simulink model "InnerTransitiontoJunction"  (R2020b)
settings: Solver=VariableStepAuto  StartTime=0.0  StopTime=10.0  RelTol=1e-3
settings Model: Creator=apple  LastModifiedBy=apple

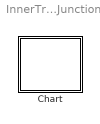
== system InnerTransitiontoJunction ==
  Chart : Stateflow chart  TreatAsAtomicUnit=on

== stateflow chart InnerTransitiontoJunction/Chart ==
  state A
    en:fprintf("Entry A");
    du:fprintf("During A");
    ex:fprintf("Exit A");
    state A1
      en:fprintf("Entry A1");
      ex:fprintf("Exit A1");
    state A2
      en:fprintf("Entry A2");
      ex:fprintf("Exit A2");
    state A3
      en:fprintf("Entry A3");
      ex:fprintf("Exit A3");
    A -> (junction 4) : E_one
    (junction 4) -> A1 [order 2] : [x > -5]
    (junction 4) -> A3 [order 3]
    (junction 4) -> A2 [order 1] : [x > -1]
    (default) -> A1
  (default) -> A : {x = 0;}
  data: x local
  events: E_one local FUNCTION_CALL_EVENT
